simulink model "unicycle_analysis"  (R2024a)
settings: Solver=VariableStepAuto  StartTime=0.0  StopTime=10.0  RelTol=1e-3
undefined symbols (not defined in the file): b_reference_point, damping_coefficient, damping_coefficient_nl, k1, k2, kp1, kp2, kp3, kp4, kv, kw, natural_frequency, natural_frequency_nl, radius
libraries: robotmobilelib x5, simulink x2
settings Model: Creator=leona  LastModifiedBy=meteh
settings DataIOCC: ReturnWorkspaceOutputsName=out1

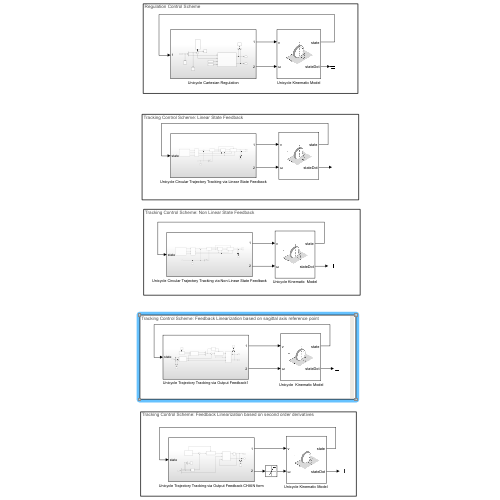
[thumbnail: Simulink's stored preview of the top-level diagram]
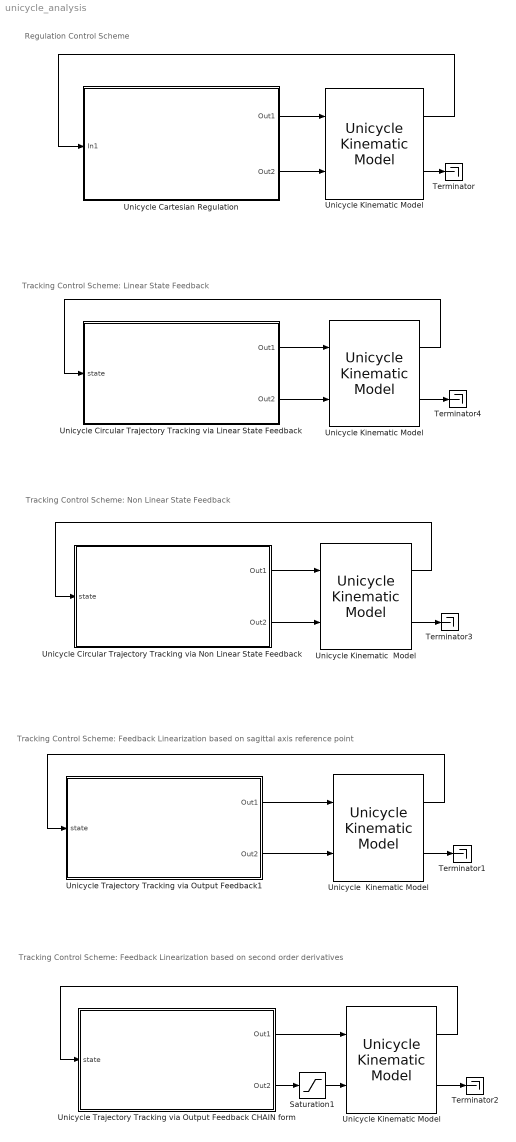
== system unicycle_analysis ==
  note: Tracking Control Scheme: Feedback Linearization based on sagittal axis reference point
  note: Tracking Control Scheme: Non Linear State Feedback
  note: Tracking Control Scheme: Linear State Feedback
  note: Tracking Control Scheme: Feedback Linearization based on second order derivatives
  note: Regulation Control Scheme
  " Unicycle  Kinematic Model" : robotmobilelib/Unicycle Kinematic Model  VehicleInputs=Vehicle Speed & Heading Angular Velocity  WheelRadius=0.01  WheelSpeedRange=[-150 150]  InitialState=[0; 0; 0]  SimulateUsing=Interpreted execution
  " Unicycle Kinematic Model " : robotmobilelib/Unicycle Kinematic Model  VehicleInputs=Vehicle Speed & Heading Angular Velocity  WheelRadius=0.01  WheelSpeedRange=[-150 150]  InitialState=[0; 0; 0]  SimulateUsing=Interpreted execution
  Saturation1 : Saturate  UpperLimit=20.5  LowerLimit=-20.5
  Terminator{,1..4} (5 alike) : Terminator
  Unicycle Cartesian Regulation : Subsystem
  Unicycle Circular Trajectory Tracking via Linear State Feedback : Subsystem
  Unicycle Circular Trajectory Tracking via Non Linear State Feedback : Subsystem
  Unicycle Kinematic  Model : robotmobilelib/Unicycle Kinematic Model  VehicleInputs=Vehicle Speed & Heading Angular Velocity  WheelRadius=0.01  WheelSpeedRange=[-150 150]  InitialState=[0; 0; 0]  SimulateUsing=Interpreted execution
  Unicycle Kinematic Model : robotmobilelib/Unicycle Kinematic Model  VehicleInputs=Vehicle Speed & Heading Angular Velocity  WheelRadius=0.01  WheelSpeedRange=[-150 150]  InitialState=[0; 0; 0]  SimulateUsing=Interpreted execution
  "Unicycle Kinematic Model " : robotmobilelib/Unicycle Kinematic Model  VehicleInputs=Vehicle Speed & Heading Angular Velocity  WheelRadius=0.01  WheelSpeedRange=[-150 150]  InitialState=[0; 0; 0]  SimulateUsing=Interpreted execution
  Unicycle Trajectory Tracking via Output Feedback CHAIN form : Subsystem
  Unicycle Trajectory Tracking via Output Feedback1 : Subsystem
  wires:
  Unicycle Cartesian Regulation/1(Out1) -> " Unicycle Kinematic Model "/1
  Unicycle Cartesian Regulation/2(Out2) -> " Unicycle Kinematic Model "/2
  " Unicycle Kinematic Model "/2 -> Terminator/1
  " Unicycle Kinematic Model "/1 -> Unicycle Cartesian Regulation/1(In1)
  Unicycle Trajectory Tracking via Output Feedback CHAIN form/1(Out1) -> "Unicycle Kinematic Model "/1
  Unicycle Trajectory Tracking via Output Feedback CHAIN form/2(Out2) -> Saturation1/1
  "Unicycle Kinematic Model "/1 -> Unicycle Trajectory Tracking via Output Feedback CHAIN form/1(state)
  "Unicycle Kinematic Model "/2 -> Terminator2/1
  Unicycle Circular Trajectory Tracking via Non Linear State Feedback/1(Out1) -> Unicycle Kinematic  Model/1
  Unicycle Circular Trajectory Tracking via Non Linear State Feedback/2(Out2) -> Unicycle Kinematic  Model/2
  Unicycle Kinematic  Model/1 -> Unicycle Circular Trajectory Tracking via Non Linear State Feedback/1(state)
  Unicycle Kinematic  Model/2 -> Terminator3/1
  Unicycle Kinematic Model/2 -> Terminator4/1
  Unicycle Circular Trajectory Tracking via Linear State Feedback/1(Out1) -> Unicycle Kinematic Model/1
  Unicycle Kinematic Model/1 -> Unicycle Circular Trajectory Tracking via Linear State Feedback/1(state)
  Unicycle Circular Trajectory Tracking via Linear State Feedback/2(Out2) -> Unicycle Kinematic Model/2
  " Unicycle  Kinematic Model"/1 -> Unicycle Trajectory Tracking via Output Feedback1/1(state)
  " Unicycle  Kinematic Model"/2 -> Terminator1/1
  Unicycle Trajectory Tracking via Output Feedback1/1(Out1) -> " Unicycle  Kinematic Model"/1
  Unicycle Trajectory Tracking via Output Feedback1/2(Out2) -> " Unicycle  Kinematic Model"/2
  Saturation1/1 -> "Unicycle Kinematic Model "/2

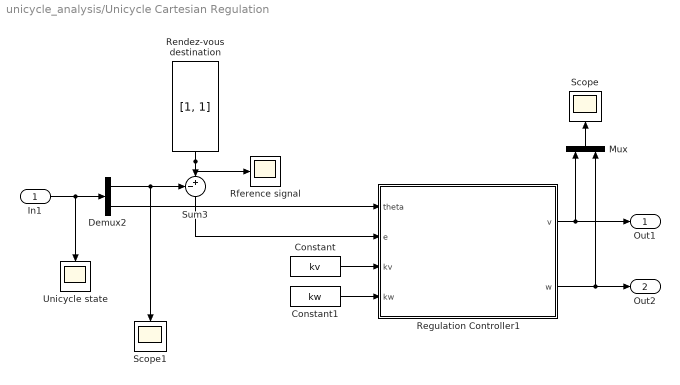
== system unicycle_analysis/Unicycle Cartesian Regulation ==
  In1 : Inport
  Constant : Constant  Value=kv
  Constant1 : Constant  Value=kw
  Demux2 : Demux  Outputs=2
  Mux : Mux  Inputs=2
  Regulation Controller1 : MATLAB Function  TreatAsAtomicUnit=on
  Rendez-vous destination : Constant  Value=[1, 1]
  Rference signal : Scope
  Scope : Scope
  Scope1 : Scope
  Sum3 : Sum  Inputs=-+|
  Unicycle state : Scope
  Out1 : Outport
  Out2 : Outport  Port=2
  wires:
  Sum3/1 -> Regulation Controller1/2(e)
  Regulation Controller1/1(v) -> Mux/1, Out1/1
  Regulation Controller1/2(w) -> Out2/1, Mux/2
  In1/1 -> Unicycle state/1, Demux2/1
  Demux2/1 -> Sum3/1, Scope1/1
  Rendez-vous destination/1 -> Rference signal/1, Sum3/2
  Demux2/2 -> Regulation Controller1/1(theta)
  Constant/1 -> Regulation Controller1/3(kv)
  Constant1/1 -> Regulation Controller1/4(kw)
  Mux/1 -> Scope/1

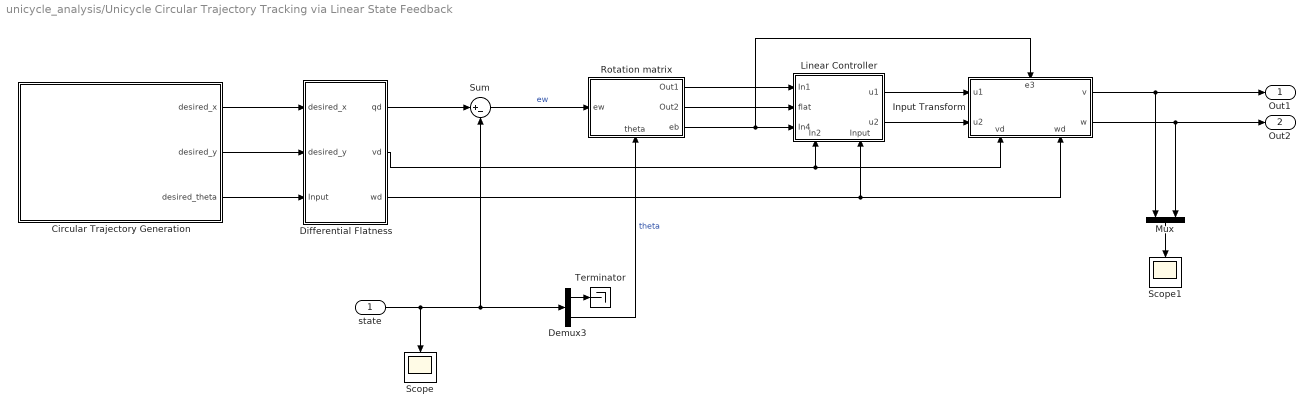
== system unicycle_analysis/Unicycle Circular Trajectory Tracking via Linear State Feedback ==
  state : Inport
  Circular Trajectory Generation : Subsystem
  Demux3 : Demux  Outputs=2
  Differential Flatness : Subsystem
  Input Transform : Subsystem
      settings: PortSchema="{\"entries\":[{\"content\":{\"sides\":[{\"content\":{\"connectorIds\":[\"In1\",\"In2\"]},\"type\":\"ConnectorPlacement.EquallySpacedRectSide\",\"uuid\":\"4380a799-56bd-42fa-b7eb-8f0915c9014b\"},{\"content\":{\"connectorIds\":[\"Out1\",\"Out2\"],\"side\":\"RIGHT\"},\"type\":\"ConnectorPlacement.EquallySpacedRectSide\",\"uuid\":\"97586fd2-c031-459c-92a6-bfbe946839f3\"},{\"content\":{\"connectorIds\":[\"In3\"],\"side\":\"TOP\"},\"type\":\"ConnectorPlacement.EquallySpacedRectSide\",\"uuid\":\"9290dd6f-8297-418b-8b82-c5c2ebc9030b\"},{\"content\":{\"connectorIds\":[\"In4\",\"In5\"],\"side\":\"BOTTOM\"},\"type\":\"ConnectorPlacement.EquallySpacedRectSide\",\"uuid\":\"808db643-f3c8-472e-94d3-d65694c039e0\"}]},\"type\":\"ConnectorPlacement.EquallySpacedConnector\",\"uuid\":\"008e5a81-0e40-4b3a-a5f3-e29ef3b642db\"}],\"packageUris\":[\"http://schema.mathworks.com/mf0/Connector/R2020b\"],\"version\":\"1.0\"}"
  Linear Controller : Subsystem
      settings: PortSchema="{\"entries\":[{\"content\":{\"sides\":[{\"content\":{\"connectorIds\":[\"In1\",\"In2\",\"In3\"]},\"type\":\"ConnectorPlacement.EquallySpacedRectSide\",\"uuid\":\"355dd5aa-d78b-48af-8d08-54ec3378b437\"},{\"content\":{\"connectorIds\":[\"Out1\",\"Out2\"],\"side\":\"RIGHT\"},\"type\":\"ConnectorPlacement.EquallySpacedRectSide\",\"uuid\":\"4abc5e76-df33-4792-8900-ee46a2dcc207\"},{\"content\":{\"side\":\"TOP\"},\"type\":\"ConnectorPlacement.EquallySpacedRectSide\",\"uuid\":\"520b05a2-b812-4ca4-b90c-01a128f1edcc\"},{\"content\":{\"connectorIds\":[\"In4\",\"In5\"],\"side\":\"BOTTOM\"},\"type\":\"ConnectorPlacement.EquallySpacedRectSide\",\"uuid\":\"7b1db8d6-e255-4c64-80bc-17cc7e8073d1\"}]},\"type\":\"ConnectorPlacement.EquallySpacedConnector\",\"uuid\":\"a570cf3a-e792-4caa-b5b1-65826e704bdc\"}],\"packageUris\":[\"http://schema.mathworks.com/mf0/Connector/R2020b\"],\"version\":\"1.0\"}"
  Mux : Mux  Inputs=2
  Rotation matrix : Subsystem
      settings: PortSchema="{\"entries\":[{\"content\":{\"sides\":[{\"content\":{\"connectorIds\":[\"In1\"]},\"type\":\"ConnectorPlacement.EquallySpacedRectSide\",\"uuid\":\"c80c5426-0069-418a-be1e-050f85102122\"},{\"content\":{\"connectorIds\":[\"Out1\",\"Out2\",\"Out3\"],\"side\":\"RIGHT\"},\"type\":\"ConnectorPlacement.EquallySpacedRectSide\",\"uuid\":\"f8dc66be-8604-4f98-b9fe-fa15c49770bc\"},{\"content\":{\"side\":\"TOP\"},\"type\":\"ConnectorPlacement.EquallySpacedRectSide\",\"uuid\":\"c5b1bfab-7e11-40da-b9ae-0f329f8970ce\"},{\"content\":{\"connectorIds\":[\"In2\"],\"side\":\"BOTTOM\"},\"type\":\"ConnectorPlacement.EquallySpacedRectSide\",\"uuid\":\"007620ed-2c8f-4927-b7e7-dbc9138b761c\"}]},\"type\":\"ConnectorPlacement.EquallySpacedConnector\",\"uuid\":\"efc411d4-2e62-4ef2-9268-9fb7a97f0e7c\"}],\"packageUris\":[\"http://schema.mathworks.com/mf0/Connector/R2020b\"],\"version\":\"1.0\"}"
  Scope : Scope
  Scope1 : Scope
  Sum : Sum  Inputs=|+-
  Terminator : Terminator
  Out1 : Outport
  Out2 : Outport  Port=2
  wires:
  Linear Controller/1(u1) -> Input Transform/1(u1)
  Linear Controller/2(u2) -> Input Transform/2(u2)
  Differential Flatness/3(wd) -> Linear Controller/5(Input), Input Transform/5(wd)
  Input Transform/1(v) -> Mux/1, Out1/1
  Differential Flatness/2(vd) -> Linear Controller/4(In2), Input Transform/4(vd)
  Differential Flatness/1(qd) -> Sum/1
  Rotation matrix/1(Out1) -> Linear Controller/1(In1)
  Sum/1 -> Rotation matrix/1(ew)  "ew"
  Input Transform/2(w) -> Out2/1, Mux/2
  state/1 -> Demux3/1, Sum/2, Scope/1
  Rotation matrix/3(eb) -> Linear Controller/3(In4), Input Transform/3(e3)
  Rotation matrix/2(Out2) -> Linear Controller/2(flat)
  Circular Trajectory Generation/1(desired_x) -> Differential Flatness/1(desired_x)
  Circular Trajectory Generation/2(desired_y) -> Differential Flatness/2(desired_y)
  Circular Trajectory Generation/3(desired_theta) -> Differential Flatness/3(Input)
  Demux3/2 -> Rotation matrix/2(theta)  "theta"
  Demux3/1 -> Terminator/1
  Mux/1 -> Scope1/1

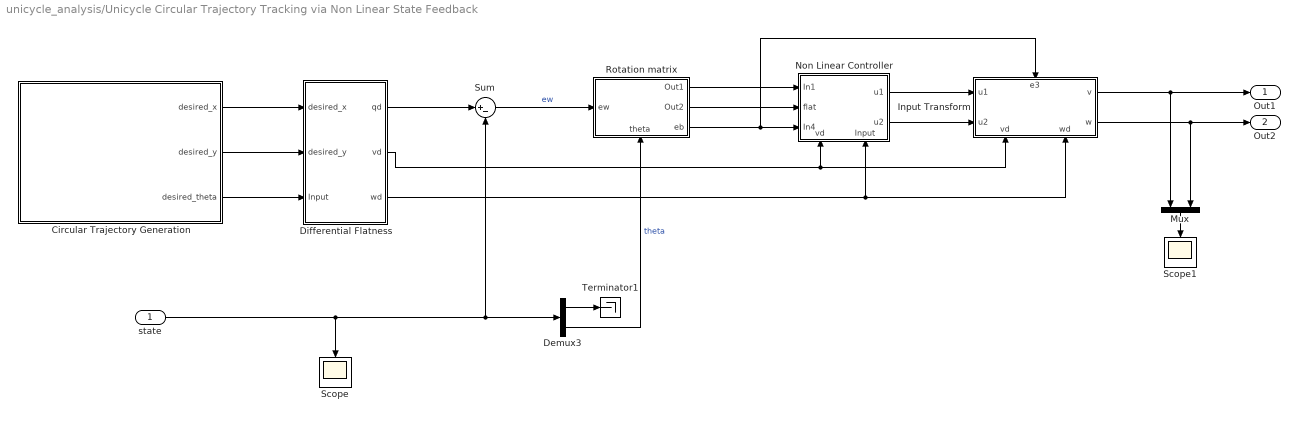
== system unicycle_analysis/Unicycle Circular Trajectory Tracking via Non Linear State Feedback ==
  state : Inport
  Circular Trajectory Generation : Subsystem
  Demux3 : Demux  Outputs=2
  Differential Flatness : Subsystem
  Input Transform : Subsystem
      settings: PortSchema="{\"entries\":[{\"content\":{\"sides\":[{\"content\":{\"connectorIds\":[\"In1\",\"In2\"]},\"type\":\"ConnectorPlacement.EquallySpacedRectSide\",\"uuid\":\"4380a799-56bd-42fa-b7eb-8f0915c9014b\"},{\"content\":{\"connectorIds\":[\"Out1\",\"Out2\"],\"side\":\"RIGHT\"},\"type\":\"ConnectorPlacement.EquallySpacedRectSide\",\"uuid\":\"97586fd2-c031-459c-92a6-bfbe946839f3\"},{\"content\":{\"connectorIds\":[\"In3\"],\"side\":\"TOP\"},\"type\":\"ConnectorPlacement.EquallySpacedRectSide\",\"uuid\":\"9290dd6f-8297-418b-8b82-c5c2ebc9030b\"},{\"content\":{\"connectorIds\":[\"In4\",\"In5\"],\"side\":\"BOTTOM\"},\"type\":\"ConnectorPlacement.EquallySpacedRectSide\",\"uuid\":\"808db643-f3c8-472e-94d3-d65694c039e0\"}]},\"type\":\"ConnectorPlacement.EquallySpacedConnector\",\"uuid\":\"008e5a81-0e40-4b3a-a5f3-e29ef3b642db\"}],\"packageUris\":[\"http://schema.mathworks.com/mf0/Connector/R2020b\"],\"version\":\"1.0\"}"
  Mux : Mux  Inputs=2
  Non Linear Controller : Subsystem
      settings: PortSchema="{\"entries\":[{\"content\":{\"sides\":[{\"content\":{\"connectorIds\":[\"In1\",\"In2\",\"In3\"]},\"type\":\"ConnectorPlacement.EquallySpacedRectSide\",\"uuid\":\"355dd5aa-d78b-48af-8d08-54ec3378b437\"},{\"content\":{\"connectorIds\":[\"Out1\",\"Out2\"],\"side\":\"RIGHT\"},\"type\":\"ConnectorPlacement.EquallySpacedRectSide\",\"uuid\":\"4abc5e76-df33-4792-8900-ee46a2dcc207\"},{\"content\":{\"side\":\"TOP\"},\"type\":\"ConnectorPlacement.EquallySpacedRectSide\",\"uuid\":\"520b05a2-b812-4ca4-b90c-01a128f1edcc\"},{\"content\":{\"connectorIds\":[\"In4\",\"In5\"],\"side\":\"BOTTOM\"},\"type\":\"ConnectorPlacement.EquallySpacedRectSide\",\"uuid\":\"7b1db8d6-e255-4c64-80bc-17cc7e8073d1\"}]},\"type\":\"ConnectorPlacement.EquallySpacedConnector\",\"uuid\":\"a570cf3a-e792-4caa-b5b1-65826e704bdc\"}],\"packageUris\":[\"http://schema.mathworks.com/mf0/Connector/R2020b\"],\"version\":\"1.0\"}"
  Rotation matrix : Subsystem
      settings: PortSchema="{\"entries\":[{\"content\":{\"sides\":[{\"content\":{\"connectorIds\":[\"In1\"]},\"type\":\"ConnectorPlacement.EquallySpacedRectSide\",\"uuid\":\"c80c5426-0069-418a-be1e-050f85102122\"},{\"content\":{\"connectorIds\":[\"Out1\",\"Out2\",\"Out3\"],\"side\":\"RIGHT\"},\"type\":\"ConnectorPlacement.EquallySpacedRectSide\",\"uuid\":\"f8dc66be-8604-4f98-b9fe-fa15c49770bc\"},{\"content\":{\"side\":\"TOP\"},\"type\":\"ConnectorPlacement.EquallySpacedRectSide\",\"uuid\":\"c5b1bfab-7e11-40da-b9ae-0f329f8970ce\"},{\"content\":{\"connectorIds\":[\"In2\"],\"side\":\"BOTTOM\"},\"type\":\"ConnectorPlacement.EquallySpacedRectSide\",\"uuid\":\"007620ed-2c8f-4927-b7e7-dbc9138b761c\"}]},\"type\":\"ConnectorPlacement.EquallySpacedConnector\",\"uuid\":\"efc411d4-2e62-4ef2-9268-9fb7a97f0e7c\"}],\"packageUris\":[\"http://schema.mathworks.com/mf0/Connector/R2020b\"],\"version\":\"1.0\"}"
  Scope : Scope
  Scope1 : Scope
  Sum : Sum  Inputs=|+-
  Terminator1 : Terminator
  Out1 : Outport
  Out2 : Outport  Port=2
  wires:
  Non Linear Controller/1(u1) -> Input Transform/1(u1)
  Non Linear Controller/2(u2) -> Input Transform/2(u2)
  Differential Flatness/3(wd) -> Non Linear Controller/5(Input), Input Transform/5(wd)
  Input Transform/1(v) -> Mux/1, Out1/1
  Differential Flatness/2(vd) -> Input Transform/4(vd), Non Linear Controller/4(vd)
  Demux3/2 -> Rotation matrix/2(theta)  "theta"
  Differential Flatness/1(qd) -> Sum/1
  Rotation matrix/1(Out1) -> Non Linear Controller/1(In1)
  Sum/1 -> Rotation matrix/1(ew)  "ew"
  Input Transform/2(w) -> Out2/1, Mux/2
  state/1 -> Scope/1, Sum/2, Demux3/1
  Rotation matrix/3(eb) -> Non Linear Controller/3(In4), Input Transform/3(e3)
  Demux3/1 -> Terminator1/1
  Rotation matrix/2(Out2) -> Non Linear Controller/2(flat)
  Circular Trajectory Generation/2(desired_y) -> Differential Flatness/2(desired_y)
  Circular Trajectory Generation/1(desired_x) -> Differential Flatness/1(desired_x)
  Circular Trajectory Generation/3(desired_theta) -> Differential Flatness/3(Input)
  Mux/1 -> Scope1/1

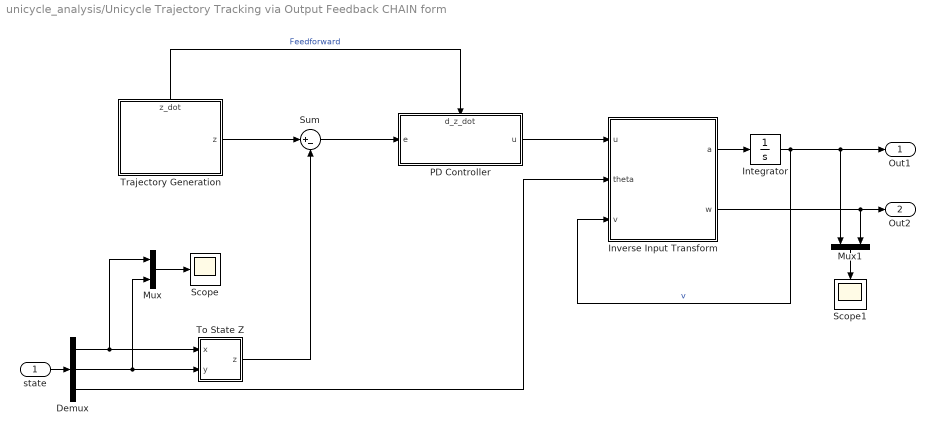
== system unicycle_analysis/Unicycle Trajectory Tracking via Output Feedback CHAIN form ==
  state : Inport
  Demux : Demux  Outputs=3
  Integrator : Integrator
  Inverse Input Transform : Subsystem
  Mux : Mux  Inputs=2
  Mux1 : Mux  Inputs=2
  PD Controller : Subsystem
      settings: PortSchema="{\"entries\":[{\"content\":{\"sides\":[{\"content\":{\"connectorIds\":[\"In1\"]},\"type\":\"ConnectorPlacement.EquallySpacedRectSide\",\"uuid\":\"55bf99ca-bf04-473b-8ad6-9178bfa9531c\"},{\"content\":{\"connectorIds\":[\"Out1\"],\"side\":\"RIGHT\"},\"type\":\"ConnectorPlacement.EquallySpacedRectSide\",\"uuid\":\"b0ca0cd6-2a6e-4bef-9c4e-2c4670ff5894\"},{\"content\":{\"connectorIds\":[\"In2\"],\"side\":\"TOP\"},\"type\":\"ConnectorPlacement.EquallySpacedRectSide\",\"uuid\":\"e96b6c80-bb25-4e2c-8bad-15410e74167e\"}]},\"type\":\"ConnectorPlacement.EquallySpacedConnector\",\"uuid\":\"4638b46a-d87f-4eb7-bee0-6d662fc14ec0\"}],\"packageUris\":[\"http://schema.mathworks.com/mf0/Connector/R2020b\"],\"version\":\"1.0\"}"
  Scope : Scope
  Scope1 : Scope
  Sum : Sum  Inputs=|+-
  To State Z : Subsystem
  Trajectory Generation : Subsystem
      settings: PortSchema="{\"entries\":[{\"content\":{\"sides\":[{\"content\":{},\"type\":\"ConnectorPlacement.EquallySpacedRectSide\",\"uuid\":\"a0648d0c-83e2-4d86-998c-15587bd2a8bf\"},{\"content\":{\"connectorIds\":[\"Out1\"],\"side\":\"RIGHT\"},\"type\":\"ConnectorPlacement.EquallySpacedRectSide\",\"uuid\":\"9fd4a5b0-b008-42bf-83da-9f9a2612716d\"},{\"content\":{\"connectorIds\":[\"Out2\"],\"side\":\"TOP\"},\"type\":\"ConnectorPlacement.EquallySpacedRectSide\",\"uuid\":\"29ce7ca0-3946-480f-b9bc-d0a41ca4b745\"}]},\"type\":\"ConnectorPlacement.EquallySpacedConnector\",\"uuid\":\"f091a176-3ac5-4616-b37c-ce46a3754a72\"}],\"packageUris\":[\"http://schema.mathworks.com/mf0/Connector/R2020b\"],\"version\":\"1.0\"}"
  Out1 : Outport
  Out2 : Outport  Port=2
  wires:
  state/1 -> Demux/1
  Demux/1 -> Mux/1, To State Z/1(x)
  Demux/2 -> Mux/2, To State Z/2(y)
  To State Z/1(z) -> Sum/2
  Sum/1 -> PD Controller/1(e)
  Integrator/1 -> Mux1/1, Out1/1, Inverse Input Transform/3(v)  "v"
  Trajectory Generation/1(z) -> Sum/1
  Trajectory Generation/2(z_dot) -> PD Controller/2(d_z_dot)  "Feedforward"
  Inverse Input Transform/1(a) -> Integrator/1
  PD Controller/1(u) -> Inverse Input Transform/1(u)
  Demux/3 -> Inverse Input Transform/2(theta)
  Inverse Input Transform/2(w) -> Mux1/2, Out2/1
  Mux/1 -> Scope/1
  Mux1/1 -> Scope1/1

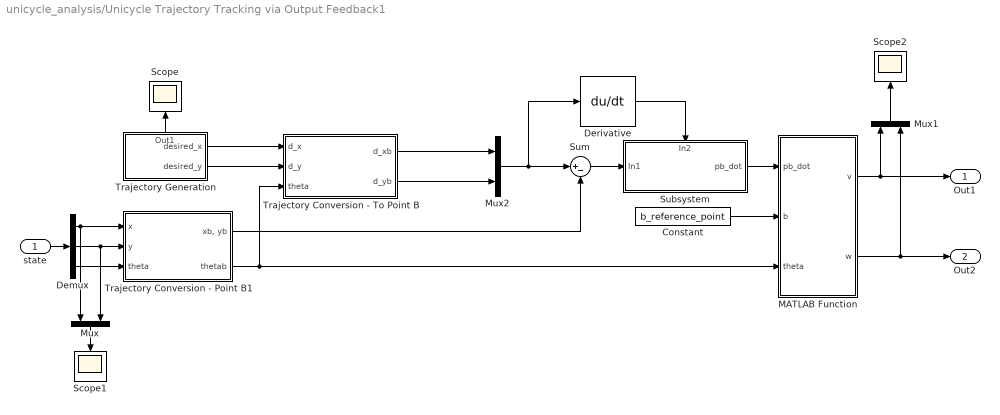
== system unicycle_analysis/Unicycle Trajectory Tracking via Output Feedback1 ==
  state : Inport
  Constant : Constant  Value=b_reference_point
  Demux : Demux  Outputs=3
  Derivative : Derivative
  MATLAB Function : MATLAB Function  TreatAsAtomicUnit=on
  Mux : Mux  Inputs=2
  Mux1 : Mux  Inputs=2
  Mux2 : Mux  Inputs=2
  Scope : Scope
  Scope1 : Scope
  Scope2 : Scope
  Subsystem : Subsystem
      settings: PortSchema="{\"entries\":[{\"content\":{\"sides\":[{\"content\":{\"connectorIds\":[\"In1\"]},\"type\":\"ConnectorPlacement.EquallySpacedRectSide\",\"uuid\":\"e1edc101-a826-4003-ad08-df84a6d82578\"},{\"content\":{\"connectorIds\":[\"Out1\"],\"side\":\"RIGHT\"},\"type\":\"ConnectorPlacement.EquallySpacedRectSide\",\"uuid\":\"f1ed9078-3db7-4a0b-b785-0b08f9ba65fc\"},{\"content\":{\"connectorIds\":[\"In2\"],\"side\":\"TOP\"},\"type\":\"ConnectorPlacement.EquallySpacedRectSide\",\"uuid\":\"e7fa8122-daf7-4fc2-869b-ae0dcfffd8f2\"}]},\"type\":\"ConnectorPlacement.EquallySpacedConnector\",\"uuid\":\"a8720b8b-968d-49c2-bed5-00f70d36dfc2\"}],\"packageUris\":[\"http://schema.mathworks.com/mf0/Connector/R2020b\"],\"version\":\"1.0\"}"
  Sum : Sum  Inputs=|+-
  Trajectory Conversion - Point B1 : Subsystem
  Trajectory Conversion - To Point B : Subsystem
  Trajectory Generation : Subsystem
      settings: PortSchema="{\"entries\":[{\"content\":{\"sides\":[{\"content\":{},\"type\":\"ConnectorPlacement.EquallySpacedRectSide\",\"uuid\":\"8d5b539f-cb35-429e-a5fa-cedc5caa952f\"},{\"content\":{\"connectorIds\":[\"Out1\",\"Out2\"],\"side\":\"RIGHT\"},\"type\":\"ConnectorPlacement.EquallySpacedRectSide\",\"uuid\":\"95bf0b02-bf52-4ab7-8c48-02064be9b571\"},{\"content\":{\"connectorIds\":[\"Out3\"],\"side\":\"TOP\"},\"type\":\"ConnectorPlacement.EquallySpacedRectSide\",\"uuid\":\"a2bfc8c2-4d82-41c7-adad-fabfe4183f1a\"}]},\"type\":\"ConnectorPlacement.EquallySpacedConnector\",\"uuid\":\"366492ce-5a31-4dd6-b5f7-03158cf0c801\"}],\"packageUris\":[\"http://schema.mathworks.com/mf0/Connector/R2020b\"],\"version\":\"1.0\"}"
  Out1 : Outport
  Out2 : Outport  Port=2
  wires:
  state/1 -> Demux/1
  Demux/1 -> Trajectory Conversion - Point B1/1(x), Mux/1
  Demux/2 -> Mux/2, Trajectory Conversion - Point B1/2(y)
  Demux/3 -> Trajectory Conversion - Point B1/3(theta)
  Trajectory Conversion - To Point B/1(d_xb) -> Mux2/1
  Trajectory Conversion - To Point B/2(d_yb) -> Mux2/2
  Mux2/1 -> Derivative/1, Sum/1
  Constant/1 -> MATLAB Function/2(b)
  Trajectory Conversion - Point B1/2(thetab) -> Trajectory Conversion - To Point B/3(theta), MATLAB Function/3(theta)
  Trajectory Generation/1(desired_x) -> Trajectory Conversion - To Point B/1(d_x)
  Trajectory Generation/2(desired_y) -> Trajectory Conversion - To Point B/2(d_y)
  Sum/1 -> Subsystem/1(In1)
  Derivative/1 -> Subsystem/2(In2)
  Subsystem/1(pb_dot) -> MATLAB Function/1(pb_dot)
  Trajectory Conversion - Point B1/1("xb, yb") -> Sum/2
  MATLAB Function/1(v) -> Mux1/1, Out1/1
  MATLAB Function/2(w) -> Out2/1, Mux1/2
  Trajectory Generation/3(Out1) -> Scope/1
  Mux/1 -> Scope1/1
  Mux1/1 -> Scope2/1

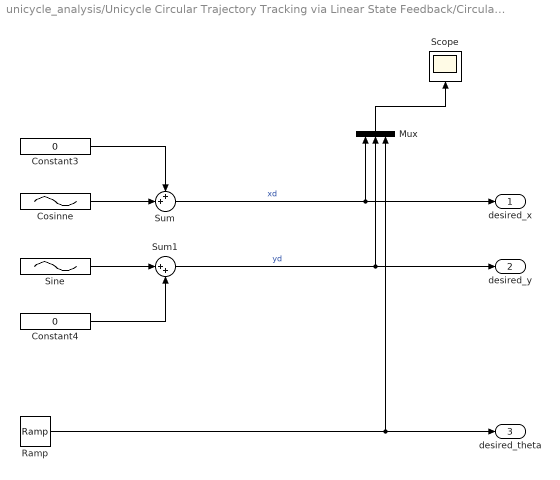
== system unicycle_analysis/Unicycle Circular Trajectory Tracking via Linear State Feedback/Circular Trajectory Generation ==
  Constant3 : Constant  Value=0
  Constant4 : Constant  Value=0
  Cosinne : Sin  Phase=pi/2  SampleTime=0
  Mux : Mux  Inputs=3
  Ramp : simulink/Sources/Ramp  slope=1  start=0  InitialOutput=pi/2
  Scope : Scope
  "Sine " : Sin  SampleTime=0
  Sum : Sum  Inputs=++|
  Sum1 : Sum  Inputs=|++
  desired_x : Outport
  desired_y : Outport  Port=2
  desired_theta : Outport  Port=3
  wires:
  Cosinne/1 -> Sum/2
  Sum/1 -> desired_x/1, Mux/1  "xd"
  Constant4/1 -> Sum1/2
  "Sine "/1 -> Sum1/1
  Sum1/1 -> desired_y/1, Mux/2  "yd"
  Constant3/1 -> Sum/1
  Mux/1 -> Scope/1
  Ramp/1 -> desired_theta/1, Mux/3

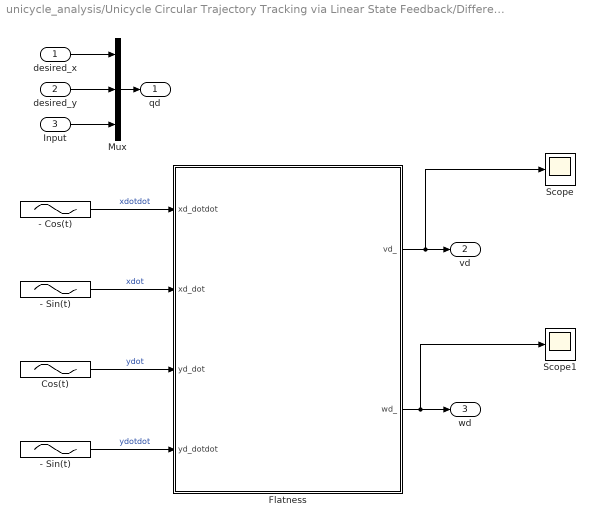
== system unicycle_analysis/Unicycle Circular Trajectory Tracking via Linear State Feedback/Differential Flatness ==
  desired_x : Inport
  desired_y : Inport  Port=2
  Input : Inport  Port=3
  - Cos(t) : Sin  Amplitude=-radius  Phase=pi/2  SampleTime=0
  - Sin(t) : Sin  Amplitude=-radius  SampleTime=0
  "- Sin(t) " : Sin  Amplitude=-radius  SampleTime=0
  "Cos(t) " : Sin  Amplitude=radius  Phase=pi/2  SampleTime=0
  Flatness : MATLAB Function  TreatAsAtomicUnit=on
  Mux : Mux  Inputs=3
  Scope : Scope
  Scope1 : Scope
  qd : Outport
  vd : Outport  Port=2
  wd : Outport  Port=3
  wires:
  Flatness/1(vd_) -> Scope/1, vd/1
  Mux/1 -> qd/1
  Flatness/2(wd_) -> Scope1/1, wd/1
  desired_y/1 -> Mux/2
  desired_x/1 -> Mux/1
  - Sin(t)/1 -> Flatness/2(xd_dot)  "xdot"
  "Cos(t) "/1 -> Flatness/3(yd_dot)  "ydot"
  "- Sin(t) "/1 -> Flatness/4(yd_dotdot)  "ydotdot"
  - Cos(t)/1 -> Flatness/1(xd_dotdot)  "xdotdot"
  Input/1 -> Mux/3

== system unicycle_analysis/Unicycle Circular Trajectory Tracking via Linear State Feedback/Input Transform ==
  u1 : Inport
  u2 : Inport  Port=2
  e3 : Inport  Port=3
  vd : Inport  Port=4
  wd : Inport  Port=5
  MATLAB Function : MATLAB Function  TreatAsAtomicUnit=on
  v : Outport
  w : Outport  Port=2
  wires:
  MATLAB Function/1(v) -> v/1
  MATLAB Function/2(w) -> w/1
  u1/1 -> MATLAB Function/1(u1)
  u2/1 -> MATLAB Function/2(u2)
  vd/1 -> MATLAB Function/3(vd)
  wd/1 -> MATLAB Function/4(wd)
  e3/1 -> MATLAB Function/5(e3)

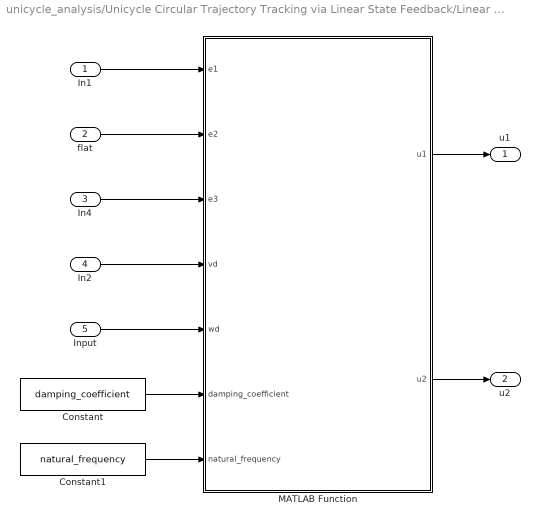
== system unicycle_analysis/Unicycle Circular Trajectory Tracking via Linear State Feedback/Linear Controller ==
  In1 : Inport
  flat : Inport  Port=2
  In4 : Inport  Port=3
  In2 : Inport  Port=4
  Input : Inport  Port=5
  Constant : Constant  Value=damping_coefficient
  Constant1 : Constant  Value=natural_frequency
  MATLAB Function : MATLAB Function  TreatAsAtomicUnit=on
  u1 : Outport
  u2 : Outport  Port=2
  wires:
  In1/1 -> MATLAB Function/1(e1)
  MATLAB Function/1(u1) -> u1/1
  MATLAB Function/2(u2) -> u2/1
  flat/1 -> MATLAB Function/2(e2)
  In4/1 -> MATLAB Function/3(e3)
  In2/1 -> MATLAB Function/4(vd)
  Input/1 -> MATLAB Function/5(wd)
  Constant/1 -> MATLAB Function/6(damping_coefficient)
  Constant1/1 -> MATLAB Function/7(natural_frequency)

== system unicycle_analysis/Unicycle Circular Trajectory Tracking via Linear State Feedback/Rotation matrix ==
  ew : Inport
  theta : Inport  Port=2
  MATLAB Function : MATLAB Function  TreatAsAtomicUnit=on
  Out1 : Outport
  Out2 : Outport  Port=2
  eb : Outport  Port=3
  wires:
  ew/1 -> MATLAB Function/1(ew)
  MATLAB Function/1(xb) -> Out1/1  "exb"
  MATLAB Function/2(yb) -> Out2/1  "eyb"
  MATLAB Function/3(thetab) -> eb/1  "ethetab"
  theta/1 -> MATLAB Function/2(theta)

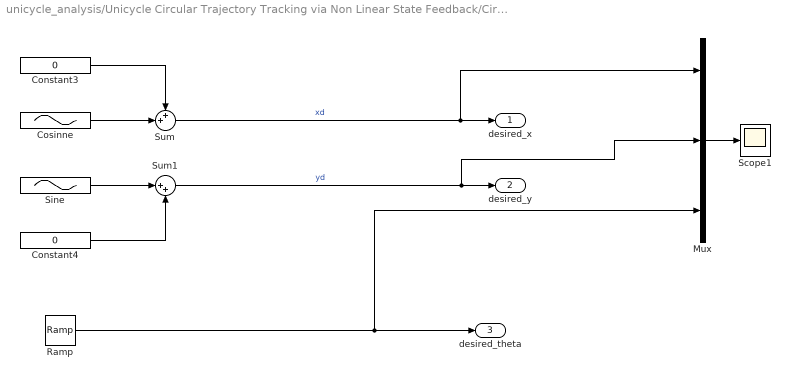
== system unicycle_analysis/Unicycle Circular Trajectory Tracking via Non Linear State Feedback/Circular Trajectory Generation ==
  Constant3 : Constant  Value=0
  Constant4 : Constant  Value=0
  Cosinne : Sin  Phase=pi/2  SampleTime=0
  Mux : Mux  Inputs=3
  Ramp : simulink/Sources/Ramp  slope=1  start=0  InitialOutput=pi/2
  Scope1 : Scope
  "Sine " : Sin  SampleTime=0
  Sum : Sum  Inputs=++|
  Sum1 : Sum  Inputs=|++
  desired_x : Outport
  desired_y : Outport  Port=2
  desired_theta : Outport  Port=3
  wires:
  Cosinne/1 -> Sum/2
  Sum/1 -> Mux/1, desired_x/1  "xd"
  Constant4/1 -> Sum1/2
  "Sine "/1 -> Sum1/1
  Sum1/1 -> Mux/2, desired_y/1  "yd"
  Constant3/1 -> Sum/1
  Mux/1 -> Scope1/1
  Ramp/1 -> Mux/3, desired_theta/1

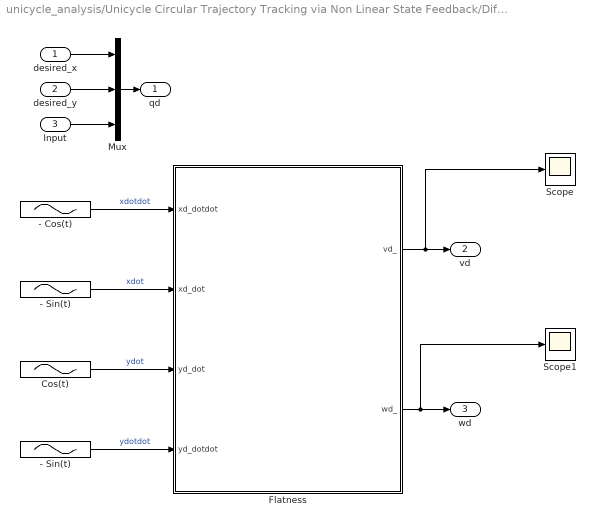
== system unicycle_analysis/Unicycle Circular Trajectory Tracking via Non Linear State Feedback/Differential Flatness ==
  desired_x : Inport
  desired_y : Inport  Port=2
  Input : Inport  Port=3
  - Cos(t) : Sin  Amplitude=-radius  Phase=pi/2  SampleTime=0
  - Sin(t) : Sin  Amplitude=-radius  SampleTime=0
  "- Sin(t) " : Sin  Amplitude=-radius  SampleTime=0
  "Cos(t) " : Sin  Amplitude=radius  Phase=pi/2  SampleTime=0
  Flatness : MATLAB Function  TreatAsAtomicUnit=on
  Mux : Mux  Inputs=3
  Scope : Scope
  Scope1 : Scope
  qd : Outport
  vd : Outport  Port=2
  wd : Outport  Port=3
  wires:
  Flatness/1(vd_) -> Scope/1, vd/1
  Mux/1 -> qd/1
  Flatness/2(wd_) -> Scope1/1, wd/1
  desired_y/1 -> Mux/2
  desired_x/1 -> Mux/1
  - Sin(t)/1 -> Flatness/2(xd_dot)  "xdot"
  "Cos(t) "/1 -> Flatness/3(yd_dot)  "ydot"
  "- Sin(t) "/1 -> Flatness/4(yd_dotdot)  "ydotdot"
  - Cos(t)/1 -> Flatness/1(xd_dotdot)  "xdotdot"
  Input/1 -> Mux/3

== system unicycle_analysis/Unicycle Circular Trajectory Tracking via Non Linear State Feedback/Input Transform ==
  u1 : Inport
  u2 : Inport  Port=2
  e3 : Inport  Port=3
  vd : Inport  Port=4
  wd : Inport  Port=5
  MATLAB Function : MATLAB Function  TreatAsAtomicUnit=on
  v : Outport
  w : Outport  Port=2
  wires:
  MATLAB Function/1(v) -> v/1
  MATLAB Function/2(w) -> w/1
  u1/1 -> MATLAB Function/1(u1)
  u2/1 -> MATLAB Function/2(u2)
  vd/1 -> MATLAB Function/3(vd)
  wd/1 -> MATLAB Function/4(wd)
  e3/1 -> MATLAB Function/5(e3)

== system unicycle_analysis/Unicycle Circular Trajectory Tracking via Non Linear State Feedback/Non Linear Controller ==
  In1 : Inport
  flat : Inport  Port=2
  In4 : Inport  Port=3
  vd : Inport  Port=4
  Input : Inport  Port=5
  Constant : Constant  Value=damping_coefficient_nl
  Constant1 : Constant  Value=natural_frequency_nl
  MATLAB Function : MATLAB Function  TreatAsAtomicUnit=on
  u1 : Outport
  u2 : Outport  Port=2
  wires:
  In1/1 -> MATLAB Function/1(e1)
  MATLAB Function/1(u1) -> u1/1
  MATLAB Function/2(u2) -> u2/1
  flat/1 -> MATLAB Function/2(e2)
  In4/1 -> MATLAB Function/3(e3)
  vd/1 -> MATLAB Function/4(vd)
  Input/1 -> MATLAB Function/5(wd)
  Constant/1 -> MATLAB Function/6(damping)
  Constant1/1 -> MATLAB Function/7(natural_frequrncy)

== system unicycle_analysis/Unicycle Circular Trajectory Tracking via Non Linear State Feedback/Rotation matrix ==
  ew : Inport
  theta : Inport  Port=2
  MATLAB Function : MATLAB Function  TreatAsAtomicUnit=on
  Out1 : Outport
  Out2 : Outport  Port=2
  eb : Outport  Port=3
  wires:
  ew/1 -> MATLAB Function/1(ew)
  MATLAB Function/1(xb) -> Out1/1  "xb"
  MATLAB Function/2(yb) -> Out2/1  "yb"
  MATLAB Function/3(thetab) -> eb/1  "thetab"
  theta/1 -> MATLAB Function/2(theta)

== system unicycle_analysis/Unicycle Trajectory Tracking via Output Feedback CHAIN form/Inverse Input Transform ==
  u : Inport
  theta : Inport  Port=2
  v : Inport  Port=3
  MATLAB Function : MATLAB Function  TreatAsAtomicUnit=on
  a : Outport
  w : Outport  Port=2
  wires:
  u/1 -> MATLAB Function/1(u)
  MATLAB Function/1(a) -> a/1
  v/1 -> MATLAB Function/3(v)
  theta/1 -> MATLAB Function/2(theta)
  MATLAB Function/2(w) -> w/1

== system unicycle_analysis/Unicycle Trajectory Tracking via Output Feedback CHAIN form/PD Controller ==
  e : Inport
  d_z_dot : Inport  Port=2
  Constant : Constant  Value=kp1
  Constant1 : Constant  Value=kp2
  Constant2 : Constant  Value=kp3
  Constant3 : Constant  Value=kp4
  MATLAB Function : MATLAB Function  TreatAsAtomicUnit=on
  Mux : Mux  Inputs=2
  u : Outport
  wires:
  e/1 -> MATLAB Function/1(e)
  d_z_dot/1 -> MATLAB Function/2(d_z_dot)
  MATLAB Function/1(u1) -> Mux/1
  MATLAB Function/2(u2) -> Mux/2
  Mux/1 -> u/1
  Constant/1 -> MATLAB Function/3(kp1_)
  Constant1/1 -> MATLAB Function/4(kp2_)
  Constant2/1 -> MATLAB Function/5(kp3_)
  Constant3/1 -> MATLAB Function/6(kp4_)

== system unicycle_analysis/Unicycle Trajectory Tracking via Output Feedback CHAIN form/To State Z ==
  x : Inport
  y : Inport  Port=2
  Derivative1 : Derivative
  Derivative2 : Derivative
  Mux : Mux
  z : Outport
  wires:
  x/1 -> Mux/1, Derivative1/1
  y/1 -> Mux/2, Derivative2/1
  Derivative1/1 -> Mux/3
  Derivative2/1 -> Mux/4
  Mux/1 -> z/1

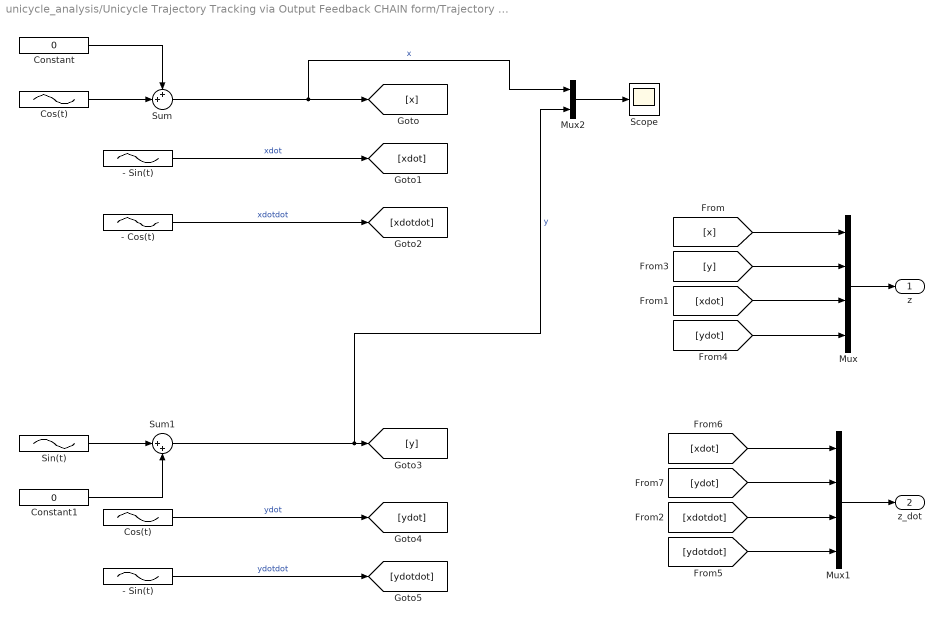
== system unicycle_analysis/Unicycle Trajectory Tracking via Output Feedback CHAIN form/Trajectory Generation ==
  - Cos(t) : Sin  Amplitude=-1  Phase=pi/2  SampleTime=0
  - Sin(t) : Sin  Amplitude=-1  SampleTime=0
  "- Sin(t) " : Sin  Amplitude=-1  SampleTime=0
  Constant : Constant  Value=0
  Constant1 : Constant  Value=0
  Cos(t) : Sin  Phase=pi/2  SampleTime=0
  "Cos(t) " : Sin  Phase=pi/2  SampleTime=0
  Mux : Mux
  Mux1 : Mux
  Mux2 : Mux  Inputs=2
  Scope : Scope
  "Sin(t) " : Sin  SampleTime=0
  Sum : Sum  Inputs=++|
  Sum1 : Sum  Inputs=|++
  z : Outport
  z_dot : Outport  Port=2
  wires:
  Cos(t)/1 -> Sum/2
  Constant/1 -> Sum/1
  Sum/1 -> Mux2/1, [x]  "x"
  "Sin(t) "/1 -> Sum1/1
  Constant1/1 -> Sum1/2
  - Sin(t)/1 -> [xdot]  "xdot"
  - Cos(t)/1 -> [xdotdot]  "xdotdot"
  Sum1/1 -> Mux2/2, [y]  "y"
  "Cos(t) "/1 -> [ydot]  "ydot"
  "- Sin(t) "/1 -> [ydotdot]  "ydotdot"
  [x] -> Mux/1
  [y] -> Mux/2
  [xdot] -> Mux/3
  [ydot] -> Mux/4
  Mux/1 -> z/1
  [xdot] -> Mux1/1
  [ydot] -> Mux1/2
  [xdotdot] -> Mux1/3
  [ydotdot] -> Mux1/4
  Mux1/1 -> z_dot/1
  Mux2/1 -> Scope/1

== system unicycle_analysis/Unicycle Trajectory Tracking via Output Feedback1/Subsystem ==
  In1 : Inport
  In2 : Inport  Port=2
  Demux1 : Demux  Outputs=2
  Gain : Gain  Gain=k1
  Gain1 : Gain  Gain=k2
  Mux : Mux  Inputs=2
  Sum : Sum  Inputs=++|
  pb_dot : Outport
  wires:
  Demux1/1 -> Gain/1
  Demux1/2 -> Gain1/1
  In1/1 -> Demux1/1
  Gain/1 -> Mux/1
  Gain1/1 -> Mux/2
  Mux/1 -> Sum/2
  In2/1 -> Sum/1
  Sum/1 -> pb_dot/1

== system unicycle_analysis/Unicycle Trajectory Tracking via Output Feedback1/Trajectory Conversion - Point B1 ==
  x : Inport
  y : Inport  Port=2
  theta : Inport  Port=3
  Constant : Constant  Value=b_reference_point
  MATLAB Function : MATLAB Function  TreatAsAtomicUnit=on
  Mux1 : Mux  Inputs=2
  "xb, yb" : Outport
  thetab : Outport  Port=2
  wires:
  x/1 -> MATLAB Function/1(x)
  y/1 -> MATLAB Function/2(y)
  theta/1 -> MATLAB Function/3(theta)
  MATLAB Function/3(thetab) -> thetab/1
  Constant/1 -> MATLAB Function/4(b)
  MATLAB Function/2(yb) -> Mux1/2
  MATLAB Function/1(xb) -> Mux1/1
  Mux1/1 -> "xb, yb"/1

== system unicycle_analysis/Unicycle Trajectory Tracking via Output Feedback1/Trajectory Conversion - To Point B ==
  d_x : Inport
  d_y : Inport  Port=2
  theta : Inport  Port=3
  Constant : Constant  Value=b_reference_point
  MATLAB Function : MATLAB Function  TreatAsAtomicUnit=on
  d_xb : Outport
  d_yb : Outport  Port=2
  wires:
  d_x/1 -> MATLAB Function/1(d_x)
  d_y/1 -> MATLAB Function/2(d_y)
  theta/1 -> MATLAB Function/3(theta)
  MATLAB Function/1(xb) -> d_xb/1
  MATLAB Function/2(yb) -> d_yb/1
  Constant/1 -> MATLAB Function/4(b)

== system unicycle_analysis/Unicycle Trajectory Tracking via Output Feedback1/Trajectory Generation ==
  Mux1 : Mux  Inputs=2
  Trajectory generation: x coordinate : Subsystem
  Trajectory generation: y coordinate : Subsystem
  desired_x : Outport
  desired_y : Outport  Port=2
  Out1 : Outport  Port=3
  wires:
  Trajectory generation: y coordinate/1(yd) -> Mux1/2, desired_y/1
  Mux1/1 -> Out1/1
  Trajectory generation: x coordinate/1(xd) -> Mux1/1, desired_x/1

== system unicycle_analysis/Unicycle Trajectory Tracking via Output Feedback1/Trajectory Generation/Trajectory generation: x coordinate ==
  Constant : Constant  Value=0
  Cosinne : Sin  Phase=pi/2  SampleTime=0
  Sum : Sum  Inputs=++|
  xd : Outport
  wires:
  Cosinne/1 -> Sum/2
  Constant/1 -> Sum/1
  Sum/1 -> xd/1  "xd"

== system unicycle_analysis/Unicycle Trajectory Tracking via Output Feedback1/Trajectory Generation/Trajectory generation: y coordinate ==
  Constant1 : Constant  Value=0
  "Sine " : Sin  SampleTime=0
  Sum1 : Sum  Inputs=|++
  yd : Outport
  wires:
  Sum1/1 -> yd/1  "yd"
  "Sine "/1 -> Sum1/1
  Constant1/1 -> Sum1/2

== matlab function unicycle_analysis/Unicycle Trajectory Tracking via Output Feedback1/MATLAB Function ==
  data: v output; pb_dot input; b input; w output; theta input
function [v, w] = fcn(pb_dot, b, theta)

    xb_dot= pb_dot(1);
    yb_dot= pb_dot(2);
    
    v= xb_dot*cos(theta) + yb_dot*sin(theta);
    
    w= xb_dot*(-sin(theta)/b) + yb_dot*(cos(theta)/b);
end

== matlab function unicycle_analysis/Unicycle Trajectory Tracking via Output Feedback1/Trajectory Conversion - Point B1/MATLAB Function ==
  data: x input; xb output; y input; theta input; yb output; thetab output; b input
function [xb, yb, thetab] = fcn(x, y, theta, b)

xb= x + b*cos(theta);
yb= y + b*sin(theta);
thetab= theta;

== matlab function unicycle_analysis/Unicycle Trajectory Tracking via Output Feedback1/Trajectory Conversion - To Point B/MATLAB Function ==
  data: d_x input; xb output; d_y input; theta input; yb output; b input
function [xb, yb] = fcn(d_x, d_y, theta, b)

xb= d_x + b*cos(theta);
yb= d_y + b*sin(theta);

== matlab function unicycle_analysis/Unicycle Trajectory Tracking via Output Feedback CHAIN form/Inverse Input Transform/MATLAB Function ==
  data: a output; u input; theta input; v input; w output
function [a, w] = fcn(u, theta, v)

    u1= u(1);
    u2= u(2);
    
    a= u1*cos(theta) + u2*sin(theta);
    
    % if the uncycle is already inside the small circle then it start with 
    % tracking and hence v=0. This implies omega to be infinite, so in this
    % case let appproximate the output w
    if v<=0.05
        w= 0.2*(u1*-theta + u2);
    else
        w= u1*(-sin(theta)/v) + u2*(cos(theta)/v);
    end
end

== matlab function unicycle_analysis/Unicycle Cartesian Regulation/Regulation Controller1 ==
  data: theta input; v output; w output; e input; kv input; kw input
function [v,w] = fcn(theta, e, kv, kw)

% evaluating if
% forward moving
% backward moving
k= sign(-(e(1)));

% linear velocity controller
v= kv*(e(1)*cos(theta) + e(2)*sin(theta));
w= kw*( atan2(-e(2), -e(1)) +(k*pi) - theta);

== matlab function unicycle_analysis/Unicycle Trajectory Tracking via Output Feedback CHAIN form/PD Controller/MATLAB Function ==
  data: e input; u1 output; d_z_dot input; u2 output; kp1_ input; kp2_ input; kp3_ input; kp4_ input
function [u1, u2] = fcn(e, d_z_dot, kp1_, kp2_, kp3_, kp4_)

    kp1= kp1_;
    kp2= kp2_;
    
    kp3= kp3_;
    kp4= kp4_;
    
    u1= kp1*(e(1)) + kp3*(e(3)) + d_z_dot(3);
    u2= kp2*(e(2)) + kp4*(e(4)) + d_z_dot(4);
end

== matlab function unicycle_analysis/Unicycle Circular Trajectory Tracking via Non Linear State Feedback/Differential Flatness/Flatness ==
  data: xd_dotdot input; xd_dot input; yd_dot input; vd_ output; wd_ output; yd_dotdot input
function [vd_, wd_] = fcn(xd_dotdot, xd_dot, yd_dot, yd_dotdot)


vd_= sqrt((xd_dot^2) + (yd_dot^2));

wd_num= (xd_dot*yd_dotdot) - (xd_dotdot*yd_dot);

wd_den= xd_dot^2 + yd_dot^2;

wd_= wd_num/wd_den;

== matlab function unicycle_analysis/Unicycle Circular Trajectory Tracking via Linear State Feedback/Differential Flatness/Flatness ==
  data: xd_dotdot input; xd_dot input; yd_dot input; vd_ output; wd_ output; yd_dotdot input
function [vd_, wd_] = fcn(xd_dotdot, xd_dot, yd_dot, yd_dotdot)


vd_= sqrt((xd_dot^2) + (yd_dot^2));

wd_num= (xd_dot*yd_dotdot) - (xd_dotdot*yd_dot);

wd_den= xd_dot^2 + yd_dot^2;

wd_= wd_num/wd_den;

== matlab function unicycle_analysis/Unicycle Circular Trajectory Tracking via Linear State Feedback/Input Transform/MATLAB Function ==
  data: u1 input; v output; u2 input; vd input; wd input; w output; e3 input
function [v, w] = fcn(u1, u2, vd, wd, e3)

    v= vd*cos(e3)- u1;
    w= wd-u2;

end

== matlab function unicycle_analysis/Unicycle Circular Trajectory Tracking via Non Linear State Feedback/Rotation matrix/MATLAB Function ==
  data: ew input; xb output; theta input; yb output; thetab output
function [xb, yb, thetab] = fcn(ew, theta)


xb=  cos(theta)*ew(1) + sin(theta)*ew(2);
yb= -sin(theta)*ew(1) + cos(theta)*ew(2);
thetab= ew(3);

== matlab function unicycle_analysis/Unicycle Circular Trajectory Tracking via Non Linear State Feedback/Input Transform/MATLAB Function ==
  data: u1 input; v output; u2 input; vd input; wd input; w output; e3 input
function [v, w] = fcn(u1, u2, vd, wd, e3)

    v= vd*cos(e3)- u1;
    w= wd-u2;
end

== matlab function unicycle_analysis/Unicycle Circular Trajectory Tracking via Linear State Feedback/Linear Controller/MATLAB Function ==
  data: e1 input; u1 output; u2 output; e2 input; e3 input; vd input; wd input; damping_coefficient input; natural_frequency input
function [u1,  u2] = fcn(e1, e2, e3, vd, wd, damping_coefficient, natural_frequency)
    
    csi= damping_coefficient;
    a= natural_frequency;
    
    k1= 2*csi*a;
    k2= (a^2 - wd^2)/vd;
    k3= k1;
    
    u1= -k1*e1;
    u2= -k2*e2 - k3*e3;

end

== matlab function unicycle_analysis/Unicycle Circular Trajectory Tracking via Linear State Feedback/Rotation matrix/MATLAB Function ==
  data: ew input; xb output; theta input; yb output; thetab output
function [xb, yb, thetab] = fcn(ew, theta)


xb=  cos(theta)*ew(1) + sin(theta)*ew(2);
yb= -sin(theta)*ew(1) + cos(theta)*ew(2);
thetab= ew(3);

== matlab function unicycle_analysis/Unicycle Circular Trajectory Tracking via Non Linear State Feedback/Non Linear Controller/MATLAB Function ==
  data: e1 input; u1 output; u2 output; e2 input; e3 input; vd input; wd input; damping input; natural_frequrncy input
function [u1,  u2] = fcn(e1, e2, e3, vd, wd, damping, natural_frequrncy)
    
    csi= damping; 
    a= natural_frequrncy;
    
    k1= 2*csi*sqrt(a*vd - wd^2);
    k3= k1;
    k2=a;
    
    u1= -k1*e1;
    u2= -k2*(vd* (sin(e3)/e3) )*e2 - (k3*e3);
end
